simulink model "ej1"  (R2023a)
settings: Solver=VariableStepAuto  StartTime=0.0  StopTime=70  MaxStep=1e-4  RelTol=1e-3
libraries: SignalEditorBlockLib x2
settings Model: Creator=Juan  LastModifiedBy=Juan

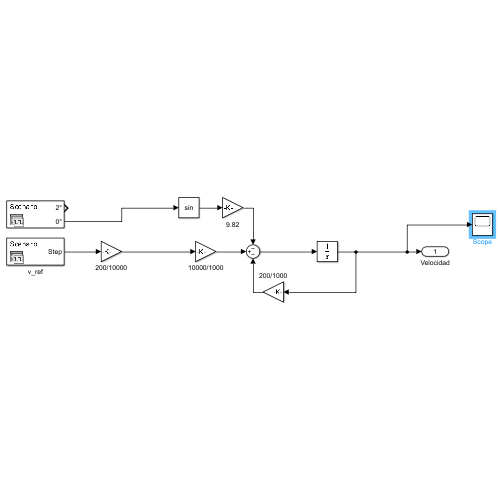
[thumbnail: Simulink's stored preview of the top-level diagram]
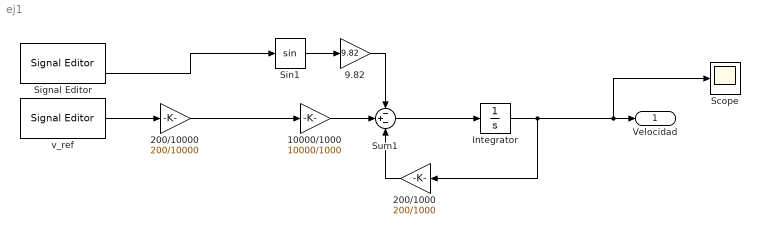
== system ej1 ==
  10000/1000 : Gain  Gain=10000/1000
  200/1000 : Gain  Gain=200/1000
  200/10000 : Gain  Gain=200/10000
  9.82 : Gain  Gain=9.82
  Integrator : Integrator  InitialCondition=25
  Scope : Scope
  Signal Editor : SignalEditorBlockLib/Signal Editor  FileName=D:\01. Facultad\Control y Sistemas1\Control y Sistemas\Tp8\perturbn.mat  ActiveScenario=Scenario  ActiveSignal=2°  IsBus=off  OutputBusObjectStr=Bus: BusObject  SampleTime=0  Interpolate=off  ZeroCross=off  OutputAfterFinalValue=Setting to zero  Unit=inherit  PreserveSignalName=on  ApplySigPropsToAllScenarios=on
  Sin1 : Trigonometry
  Sum1 : Sum  Inputs=-+-
  v_ref : SignalEditorBlockLib/Signal Editor  FileName=D:\01. Facultad\Control y Sistemas1\Control y Sistemas\Tp8\v_ref.mat  ActiveScenario=Scenario  ActiveSignal=Step  IsBus=off  OutputBusObjectStr=Bus: BusObject  SampleTime=0  Interpolate=off  ZeroCross=off  OutputAfterFinalValue=Setting to zero  Unit=inherit  PreserveSignalName=on  ApplySigPropsToAllScenarios=on
  Velocidad : Outport
  wires:
  v_ref/1 -> 200/10000/1
  200/10000/1 -> 10000/1000/1
  Signal Editor/2 -> Sin1/1
  Sin1/1 -> 9.82/1
  9.82/1 -> Sum1/1
  200/1000/1 -> Sum1/3
  Sum1/1 -> Integrator/1
  Integrator/1 -> 200/1000/1, Scope/1, Velocidad/1
  10000/1000/1 -> Sum1/2
